simulink model "aircraft_pitch_control"  (R2017a)
settings: Solver=ode45  StartTime=0.0  StopTime=10.0  RelTol=1e-3
settings Model: Creator=sansh  LastModifiedBy=sansh

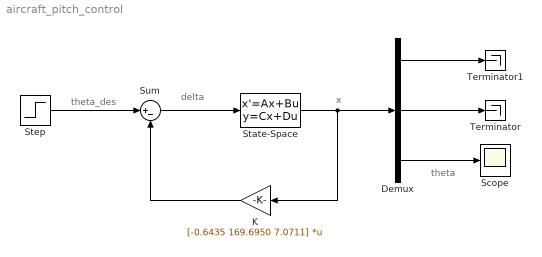
== system aircraft_pitch_control ==
  note: theta
  note: x
  note: theta_des
  note: delta
  Demux : Demux  Outputs=3
  K : Gain  Gain=[-0.6435 169.6950 7.0711]  Multiplication=Matrix(K*u)
  Scope : Scope
  State-Space : StateSpace  A=[-0.313 56.7 0; -0.0139 -0.426 0; 0 56.7 0]  B=[0.232; 0.0203; 0]  C=eye(3)  D=[0;0;0]  X0=0  ContinuousStateAttributes={'Angle_of_attack','Pitch_rate','Pitch_angle'}
  Step : Step  Time=0  After=0.2  SampleTime=0
  Sum : Sum  Inputs=|+-
  Terminator : Terminator
  Terminator1 : Terminator
  wires:
  Demux/2 -> Terminator/1
  Demux/1 -> Terminator1/1
  State-Space/1 -> K/1, Demux/1
  Demux/3 -> Scope/1
  Sum/1 -> State-Space/1
  Step/1 -> Sum/1
  K/1 -> Sum/2
